simulink model "BLDC_system_diagram"  (R2013a)
settings: Solver=ode45  StartTime=0.0  StopTime=0.5  RelTol=1e-3
undefined symbols (not defined in the file or in its folder): Accelerationmax, Accelerationmin, DiscIntNeverNeededParam, IDCmax, IDCmin, Iphasepeakmax, P, PM, Risetimemax, Speedmax, Stalltimemax, Temperaturemax, Ts, VDCmax, VDCmin, VDCrated
undefined symbols (not defined in the file): Rs
libraries: simulink x68, powerlib_meascontrol x9, spsPMSynchronousMachineModel x3, simulink_extras x2
(part 1 of 3)
settings Model: Creator=Sony  LastModifiedBy=Muhammad Shamaas

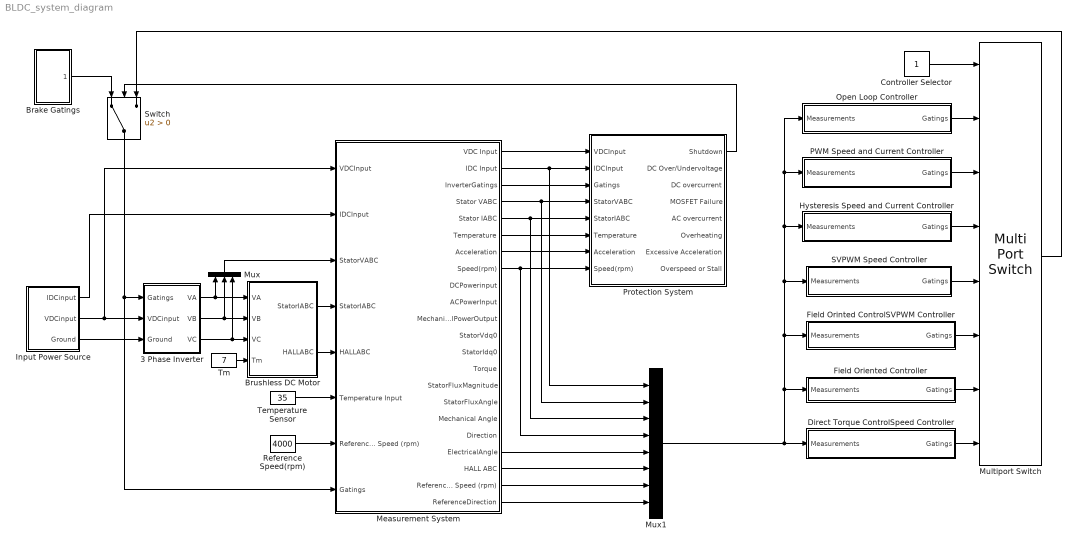
== system BLDC_system_diagram ==
  " Field Orinted ControlSVPWM Controller" : Subsystem
  3 Phase Inverter : Subsystem
  Brake Gatings : Subsystem
  Brushless DC Motor : Subsystem
  Controller Selector : Constant
  Direct Torque ControlSpeed Controller : Subsystem
  Field Oriented Controller : Subsystem
  Hysteresis Speed and Current Controller : Subsystem
  Input Power Source : Subsystem
  Measurement System : Subsystem
  Multiport Switch : MultiPortSwitch  Inputs=7
  Mux : Mux  Inputs=3
  Mux1 : Mux  Inputs=8
  Open Loop Controller : Subsystem
  PWM Speed and Current Controller : Subsystem
  Protection System : Subsystem
  Reference Speed(rpm) : Constant  Value=4000
  SVPWM Speed Controller : Subsystem
  Switch : Switch  Criteria=u2 > Threshold
  Temperature Sensor : Constant  Value=35
  Tm : Constant  Value=7
  wires:
  Input Power Source/2(VDCinput) -> Measurement System/1(VDCInput), 3 Phase Inverter/2(VDCinput)
  Input Power Source/3(Ground) -> 3 Phase Inverter/3(Ground)
  3 Phase Inverter/1(VA) -> Brushless DC Motor/1(VA), Mux/1
  3 Phase Inverter/2(VB) -> Brushless DC Motor/2(VB), Mux/2
  Brushless DC Motor/2(HALLABC) -> Measurement System/5(HALLABC)
  Brushless DC Motor/1(StatorIABC) -> Measurement System/4(StatorIABC)
  Mux/1 -> Measurement System/3(StatorVABC)
  3 Phase Inverter/3(VC) -> Brushless DC Motor/3(VC), Mux/3
  Measurement System/8(Speed(rpm)) -> Mux1/4, Protection System/8(Speed(rpm))
  Measurement System/7(Acceleration) -> Protection System/7(Acceleration)
  Measurement System/6(Temperature) -> Protection System/6(Temperature)
  Measurement System/5(Stator IABC) -> Mux1/3, Protection System/5(StatorIABC)
  Measurement System/4(Stator VABC) -> Mux1/2, Protection System/4(StatorVABC)
  Measurement System/3(InverterGatings) -> Protection System/3(Gatings)
  Measurement System/1(VDC Input) -> Protection System/1(VDCInput)
  Switch/1 -> Measurement System/8(Gatings), 3 Phase Inverter/1(Gatings)
  Multiport Switch/1 -> Switch/3
  Protection System/1(Shutdown) -> Switch/2
  Controller Selector/1 -> Multiport Switch/1
  Measurement System/2(IDC Input) -> Mux1/1, Protection System/2(IDCInput)
  Mux1/1 -> Field Oriented Controller/1(Measurements), " Field Orinted ControlSVPWM Controller"/1(Measurements), SVPWM Speed Controller/1(Measurements), Open Loop Controller/1(Measurements), PWM Speed and Current Controller/1(Measurements), Hysteresis Speed and Current Controller/1(Measurements), Direct Torque ControlSpeed Controller/1(Measurements)
  Measurement System/22(ReferenceDirection) -> Mux1/8
  Measurement System/21(Reference Speed (rpm)) -> Mux1/7
  Measurement System/20(HALL ABC) -> Mux1/6
  Measurement System/19(ElectricalAngle) -> Mux1/5
  Reference Speed(rpm)/1 -> Measurement System/7(Reference Speed (rpm))
  Brake Gatings/1(Gatings) -> Switch/1
  Open Loop Controller/1(Gatings) -> Multiport Switch/2
  PWM Speed and Current Controller/1(Gatings) -> Multiport Switch/3
  Hysteresis Speed and Current Controller/1(Gatings) -> Multiport Switch/4
  SVPWM Speed Controller/1(Gatings) -> Multiport Switch/5
  " Field Orinted ControlSVPWM Controller"/1(Gatings) -> Multiport Switch/6
  Field Oriented Controller/1(Gatings) -> Multiport Switch/7
  Direct Torque ControlSpeed Controller/1(Gatings) -> Multiport Switch/8
  Input Power Source/1(IDCinput) -> Measurement System/2(IDCInput)
  Temperature Sensor/1 -> Measurement System/6(Temperature Input)
  Tm/1 -> Brushless DC Motor/4(Tm)

== system BLDC_system_diagram/ Field Orinted ControlSVPWM Controller ==
  Measurements : Inport
  " Field Orinted ControlSVPWM Controller" : Subsystem
  Fcn14 : Fcn  Expr=u(5)
  Fcn15 : Fcn  Expr=u(7)
  Fcn16 : Fcn  Expr=u(3)
  Fcn17 : Fcn  Expr=u(4)
  Gatings : Outport
  wires:
  " Field Orinted ControlSVPWM Controller"/1(Gatings) -> Gatings/1
  Fcn14/1 -> " Field Orinted ControlSVPWM Controller"/4(Thetae)
  Fcn17/1 -> " Field Orinted ControlSVPWM Controller"/1(RotorSpeed(rpm))
  Fcn16/1 -> " Field Orinted ControlSVPWM Controller"/2(Iabc)
  Fcn15/1 -> " Field Orinted ControlSVPWM Controller"/3(ReferenceRotorSpeed(rpm))
  Measurements/1 -> Fcn14/1, Fcn15/1, Fcn17/1, Fcn16/1

== system BLDC_system_diagram/3 Phase Inverter ==
  note: Three Phase Inverter
      | HighSideGateSignal       LowSideGateSignal       Output
      | 0                                  0                 undefined
      | 0                                  1                    Ground
      | 1                                  0                 VDCInput
      | 1                                  1                   undefined
  Gatings : Inport
  VDCinput : Inport  Port=2
  Ground : Inport  Port=3
  Average : Subsystem
  Average1 : Subsystem
  Average2 : Subsystem
  Demux : Demux  Outputs=6
  Switch{,1..5} (6 alike) : Switch
  VA : Outport
  VB : Outport  Port=2
  VC : Outport  Port=3
  wires:
  [s1] -> Switch/2
  Demux/1 -> [s1]
  Demux/2 -> [s2]
  Demux/3 -> [s3]
  Demux/4 -> [s4]
  Demux/5 -> [s5]
  Demux/6 -> [s6]
  Gatings/1 -> Demux/1
  [s2] -> Switch3/2
  VDCinput/1 -> Switch/1, Switch5/1, Switch4/1
  Switch/1 -> Average/1(In1)
  Switch3/1 -> Average/2(In2)
  Average/1(Out1) -> VA/1
  Average1/1(Out1) -> VB/1
  Average2/1(Out1) -> VC/1
  [s4] -> Switch1/2
  [s6] -> Switch2/2
  Ground/1 -> Switch3/1, Switch2/1, Switch1/1
  [s3] -> Switch4/2
  [s5] -> Switch5/2
  Switch4/1 -> Average1/1(In1)
  Switch1/1 -> Average1/2(In2)
  Switch2/1 -> Average2/2(In2)
  Switch5/1 -> Average2/1(In1)

== system BLDC_system_diagram/Brake Gatings ==
  Brake Gatings : Constant  Value=[0;0;0]
  Compare To Zero : simulink/Logic and Bit Operations/Compare To Zero  relop=>=  OutDataTypeStr=boolean
  Constant : Constant  Value=0
  Gates : Subsystem
  Sum2 : Sum  Inputs=|+-
  TRI : powerlib_meascontrol/Pulse & Signal Generators/Triangle Generator  Freq=1e4  Phase=0  Ts=0
  Gatings : Outport
  wires:
  Compare To Zero/1 -> Gates/2(PWM)
  Gates/1(Gates) -> Gatings/1
  Sum2/1 -> Compare To Zero/1
  TRI/1 -> Sum2/2
  Brake Gatings/1 -> Gates/1("emf_abc ")
  Constant/1 -> Sum2/1

== system BLDC_system_diagram/Brushless DC Motor ==
  VA : Inport
  VB : Inport  Port=2
  VC : Inport  Port=3
  Tm : Inport  Port=4
  Add : Sum  Inputs=+-
  Add1 : Sum  Inputs=+-
  Electrical Model : Subsystem
  Mechanical Model : Subsystem
  Mux : Mux  Inputs=2
  Mux1 : Mux  Inputs=3
  Mux2 : Mux  Inputs=3
  Subsystem : Subsystem
  StatorIABC : Outport
  HALLABC : Outport  Port=2
  wires:
  Tm/1 -> Mechanical Model/1(Tm)
  Add/1 -> Mux/1
  Add1/1 -> Mux/2
  Mux/1 -> Electrical Model/1(v)  "vab,vbc"
  Electrical Model/1(m) -> Subsystem/1(m_e)
  Mechanical Model/2(the) -> Electrical Model/3(the)
  VB/1 -> Add1/1, Add/2
  VC/1 -> Add1/2
  Mechanical Model/1(we) -> Electrical Model/2(we)
  Electrical Model/2(Te) -> Mechanical Model/2(Te)
  Mechanical Model/3(m) -> Subsystem/2(m_m)
  VA/1 -> Add/1
  Subsystem/1(Stator current is_a (A)) -> Mux1/1
  Subsystem/2(Stator current is_b (A)) -> Mux1/2
  Subsystem/3(Stator current is_c (A)) -> Mux1/3
  Subsystem/4(Hall effect signal h_a) -> Mux2/1
  Subsystem/5(Hall effect signal h_b) -> Mux2/2
  Subsystem/6(Hall effect signal h_c) -> Mux2/3
  Mux2/1 -> HALLABC/1
  Mux1/1 -> StatorIABC/1

== system BLDC_system_diagram/Direct Torque ControlSpeed Controller ==
  Measurements : Inport
  Direct Torque ControlSpeed Controller : Subsystem
  Fcn22 : Fcn  Expr=u(7)
  Fcn23 : Fcn  Expr=u(4)
  Fcn24 : Fcn  Expr=u(3)
  Fcn25 : Fcn  Expr=u(2)
  Gatings : Outport
  wires:
  Direct Torque ControlSpeed Controller/1(Gatings) -> Gatings/1
  Fcn22/1 -> Direct Torque ControlSpeed Controller/4(ReferenceRotorSpeed(rpm))
  Fcn23/1 -> Direct Torque ControlSpeed Controller/3(RotorSpeed(rpm))
  Fcn24/1 -> Direct Torque ControlSpeed Controller/2(StatorIABC)
  Fcn25/1 -> Direct Torque ControlSpeed Controller/1(StatorVABC)
  Measurements/1 -> Fcn22/1, Fcn23/1, Fcn25/1, Fcn24/1

== system BLDC_system_diagram/Field Oriented Controller ==
  Measurements : Inport
  Fcn18 : Fcn  Expr=u(7)
  Fcn19 : Fcn  Expr=u(5)
  Fcn20 : Fcn  Expr=u(4)
  Fcn21 : Fcn  Expr=u(3)
  Field Oriented Control Current and Speed Controller : Subsystem
  Gatings : Outport
  wires:
  Field Oriented Control Current and Speed Controller/1(Gatings) -> Gatings/1
  Fcn20/1 -> Field Oriented Control Current and Speed Controller/2(RotorSpeed(rpm))
  Fcn19/1 -> Field Oriented Control Current and Speed Controller/3(Rotor Electrical Angle)
  Fcn21/1 -> Field Oriented Control Current and Speed Controller/1(Stator IABC)
  Fcn18/1 -> Field Oriented Control Current and Speed Controller/4(ReferenceRotorSpeed(rpm))
  Measurements/1 -> Fcn18/1, Fcn19/1, Fcn21/1, Fcn20/1

== system BLDC_system_diagram/Hysteresis Speed and Current Controller ==
  Measurements : Inport
  Fcn10 : Fcn  Expr=u(6)
  Fcn7 : Fcn  Expr=u(7)
  Fcn8 : Fcn  Expr=u(4)
  Fcn9 : Fcn  Expr=u(3)
  Hysteresis Speed and Current Controller : Subsystem
  Gatings : Outport
  wires:
  Measurements/1 -> Fcn7/1, Fcn8/1, Fcn10/1, Fcn9/1
  Fcn10/1 -> Hysteresis Speed and Current Controller/1(HALLABC)
  Hysteresis Speed and Current Controller/1(Gatings) -> Gatings/1
  Fcn8/1 -> Hysteresis Speed and Current Controller/3(RotorSpeed(rpm))
  Fcn7/1 -> Hysteresis Speed and Current Controller/4(ReferenceRotorSpeed(rpm))
  Fcn9/1 -> Hysteresis Speed and Current Controller/2(StatorIABC)

== system BLDC_system_diagram/Input Power Source ==
  IDCinput : Outport
  VDCinput : Outport  Port=2
  Ground : Outport  Port=3

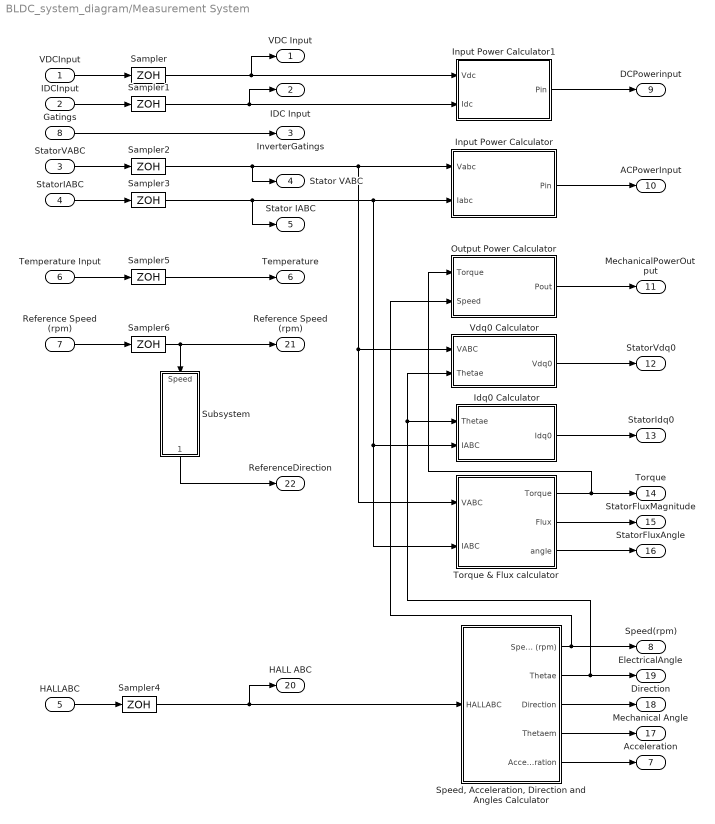
== system BLDC_system_diagram/Measurement System ==
  VDCInput : Inport
  IDCInput : Inport  Port=2
  StatorVABC : Inport  Port=3
  StatorIABC : Inport  Port=4
  HALLABC : Inport  Port=5
  Temperature Input : Inport  Port=6
  Reference Speed (rpm) : Inport  Port=7
  Gatings : Inport  Port=8
  Idq0 Calculator : Subsystem
  Input Power Calculator : Subsystem
  Input Power Calculator1 : Subsystem
  Output Power Calculator : Subsystem
  Sampler{,1..6} (7 alike) : ZeroOrderHold  SampleTime=1e-4
  "Speed, Acceleration, Direction and Angles Calculator" : Subsystem
  Subsystem : Subsystem
  Torque & Flux calculator : Subsystem  AncestorBlock=electricdrivelib/AC drives/DTC Induction Motor Drive/DTC/Torque & Flux calculator  mask{Rss=Rs, P=P, Ts=Ts}
  Vdq0 Calculator : Subsystem
  VDC Input : Outport
  IDC Input : Outport  Port=2
  InverterGatings : Outport  Port=3
  Stator VABC : Outport  Port=4
  Stator IABC : Outport  Port=5
  Temperature : Outport  Port=6
  Acceleration : Outport  Port=7
  Speed(rpm) : Outport  Port=8
  DCPowerinput : Outport  Port=9
  ACPowerInput : Outport  Port=10
  MechanicalPowerOutput : Outport  Port=11
  StatorVdq0 : Outport  Port=12
  StatorIdq0 : Outport  Port=13
  Torque : Outport  Port=14
  StatorFluxMagnitude : Outport  Port=15
  StatorFluxAngle : Outport  Port=16
  Mechanical Angle : Outport  Port=17
  Direction : Outport  Port=18
  ElectricalAngle : Outport  Port=19
  HALL ABC : Outport  Port=20
  Reference Speed (rpm) : Outport  Port=21
  ReferenceDirection : Outport  Port=22
  wires:
  HALLABC/1 -> Sampler4/1
  Sampler/1 -> VDC Input/1, Input Power Calculator1/1(Vdc)
  IDCInput/1 -> Sampler1/1
  "Speed, Acceleration, Direction and Angles Calculator"/2(Thetae) -> ElectricalAngle/1, Idq0 Calculator/1(Thetae), Vdq0 Calculator/2(Thetae)
  StatorIABC/1 -> Sampler3/1
  Torque & Flux calculator/1(Torque) -> Torque/1, Output Power Calculator/1(Torque)
  StatorVABC/1 -> Sampler2/1
  "Speed, Acceleration, Direction and Angles Calculator"/1(Speed (rpm)) -> Output Power Calculator/2(Speed), Speed(rpm)/1
  Input Power Calculator1/1(Pin) -> DCPowerinput/1
  Torque & Flux calculator/3(angle) -> StatorFluxAngle/1
  "Speed, Acceleration, Direction and Angles Calculator"/5(Acceleration) -> Acceleration/1
  Output Power Calculator/1(Pout) -> MechanicalPowerOutput/1
  Idq0 Calculator/1(Idq0) -> StatorIdq0/1
  "Speed, Acceleration, Direction and Angles Calculator"/3(Direction) -> Direction/1
  Input Power Calculator/1(Pin) -> ACPowerInput/1
  Vdq0 Calculator/1(Vdq0) -> StatorVdq0/1
  "Speed, Acceleration, Direction and Angles Calculator"/4(Thetaem) -> Mechanical Angle/1
  Torque & Flux calculator/2(Flux) -> StatorFluxMagnitude/1
  VDCInput/1 -> Sampler/1
  Sampler1/1 -> IDC Input/1, Input Power Calculator1/2(Idc)
  Sampler2/1 -> Stator VABC/1, Torque & Flux calculator/1(VABC), Vdq0 Calculator/1(VABC), Input Power Calculator/1(Vabc)
  Sampler3/1 -> Stator IABC/1, Torque & Flux calculator/2(IABC), Idq0 Calculator/2(IABC), Input Power Calculator/2(Iabc)
  Sampler4/1 -> HALL ABC/1, "Speed, Acceleration, Direction and Angles Calculator"/1(HALLABC)
  Temperature Input/1 -> Sampler5/1
  Sampler5/1 -> Temperature/1
  Reference Speed (rpm)/1 -> Sampler6/1
  Sampler6/1 -> Subsystem/1(Speed), Reference Speed (rpm)/1
  Gatings/1 -> InverterGatings/1
  Subsystem/1(Direction) -> ReferenceDirection/1

== system BLDC_system_diagram/Open Loop Controller ==
  Measurements : Inport
  Fcn : Fcn  Expr=u(6)
  Fcn1 : Fcn  Expr=u(8)
  Open Loop Controller : Subsystem
  Gatings : Outport
  wires:
  Open Loop Controller/1(Gatings) -> Gatings/1
  Fcn1/1 -> Open Loop Controller/2(Direction)
  Fcn/1 -> Open Loop Controller/1(HALLSensorABCSignals)
  Measurements/1 -> Fcn1/1, Fcn/1

== system BLDC_system_diagram/PWM Speed and Current Controller ==
  Measurements : Inport
  Fcn2 : Fcn  Expr=u(7)
  Fcn4 : Fcn  Expr=u(4)
  Fcn5 : Fcn  Expr=u(1)
  Fcn6 : Fcn  Expr=u(6)
  PWM Speed and Current Controller : Subsystem
  Gatings : Outport
  wires:
  Fcn6/1 -> PWM Speed and Current Controller/1(HALLABC)
  Fcn5/1 -> PWM Speed and Current Controller/2(IDCInput)
  Fcn4/1 -> PWM Speed and Current Controller/3(RotorSpeed(rpm))
  Fcn2/1 -> PWM Speed and Current Controller/4(ReferenceRotorSpeed(rpm))
  PWM Speed and Current Controller/1(Gatings) -> Gatings/1
  Measurements/1 -> Fcn2/1, Fcn4/1, Fcn6/1, Fcn5/1

== system BLDC_system_diagram/Protection System ==
  VDCInput : Inport
  IDCInput : Inport  Port=2
  Gatings : Inport  Port=3
  StatorVABC : Inport  Port=4
  StatorIABC : Inport  Port=5
  Temperature : Inport  Port=6
  Acceleration : Inport  Port=7
  Speed(rpm) : Inport  Port=8
  AC overcurrent Protection : Subsystem
  DC Over/Undervoltage Protection : Subsystem
  DC overcurrent Protection : Subsystem
  Excessive Acceleration/Deceleration Protection : Subsystem
  Logical Operator : Logic  Operator=OR  Inputs=7  AllPortsSameDT=off  OutDataTypeStr=boolean
  MOSFET Failure Protection : Subsystem
  Overheating Protection : Subsystem
  Overspeed and Stall Protection : Subsystem
  Shutdown : Outport
  DC Over/Undervoltage : Outport  Port=2
  DC overcurrent : Outport  Port=3
  MOSFET Failure : Outport  Port=4
  AC overcurrent : Outport  Port=5
  Overheating : Outport  Port=6
  Excessive Acceleration : Outport  Port=7
  Overspeed or Stall : Outport  Port=8
  tag scope: Shutdown=global
  wires:
  AC overcurrent Protection/1(Out1) -> Logical Operator/4, AC overcurrent/1
  DC overcurrent Protection/1(Out1) -> Logical Operator/2, DC overcurrent/1
  DC Over/Undervoltage Protection/1(Out1) -> Logical Operator/1, DC Over/Undervoltage/1
  Overheating Protection/1(Out1) -> Logical Operator/5, Overheating/1
  MOSFET Failure Protection/1(Out1) -> Logical Operator/3, MOSFET Failure/1
  Excessive Acceleration/Deceleration Protection/1(Out1) -> Logical Operator/6, Excessive Acceleration/1
  Overspeed and Stall Protection/1(Out1) -> Logical Operator/7, Overspeed or Stall/1
  Logical Operator/1 -> [Shutdown], Shutdown/1
  VDCInput/1 -> DC Over/Undervoltage Protection/1(VDC)
  IDCInput/1 -> DC overcurrent Protection/1(IDCInput)
  Gatings/1 -> MOSFET Failure Protection/1(Gatings)
  StatorVABC/1 -> MOSFET Failure Protection/2(StatorVABC)
  StatorIABC/1 -> AC overcurrent Protection/1(StatorIABC)
  Temperature/1 -> Overheating Protection/1(Temperature)
  Acceleration/1 -> Excessive Acceleration/Deceleration Protection/1(Acceleration)
  Speed(rpm)/1 -> Overspeed and Stall Protection/1(Speed(rpm))

== system BLDC_system_diagram/SVPWM Speed Controller ==
  Measurements : Inport
  Fcn11 : Fcn  Expr=u(7)
  Fcn12 : Fcn  Expr=u(4)
  Fcn13 : Fcn  Expr=u(6)
  SVPWM Speed Controller : Subsystem
  Gatings : Outport
  wires:
  SVPWM Speed Controller/1(Gatings) -> Gatings/1
  Fcn13/1 -> SVPWM Speed Controller/1(HALLABC)
  Fcn12/1 -> SVPWM Speed Controller/2(RotorSpeed(rpm))
  Fcn11/1 -> SVPWM Speed Controller/3(ReferenceRotorSpeed(rpm))
  Measurements/1 -> Fcn11/1, Fcn13/1, Fcn12/1

== system BLDC_system_diagram/ Field Orinted ControlSVPWM Controller/ Field Orinted ControlSVPWM Controller ==
  note: void writestate (int sa, int sb, int sc)
      | {
      |   if (sa==1)    {digitalWrite(PhaseaUpperPin, HIGH);digitalWrite(PhaseaLowerPin, LOW);}
      |   if (sa==(-1)){digitalWrite(PhaseaUpperPin, LOW) ;digitalWrite(PhaseaLowerPin, HIGH);}
      |   if (sa==0)    {digitalWrite(PhaseaUpperPin, LOW) ;digitalWrite(PhaseaLowerPin, LOW);}
      |   if (sb==1)    {digitalWrite(PhasebUpperPin, HIGH);digitalWrite(PhasebLowerPin, LOW);}
      |   if (sb==(-1)){digitalWrite(PhasebUpperPin, LOW) ;digitalWrite(PhasebLowerPin, HIGH);}
      |   if (sb==0)    {digitalWrite(PhasebUpperPin, LOW) ;digitalWrite(PhasebLowerPin, LOW);}
      |   if (sc==1)    {digitalWrite(PhasecUpperPin, HIGH);digitalWrite(PhasecLowerPin, LOW);}
      |   if (sc==(-1)){digitalWrite(PhasecUpperPin, LOW) ;digitalWrite(PhasecLowerPin, HIGH);}
      |   if (sc==0)    {digitalWrite(PhasecUpperPin, LOW) ;digitalWrite(PhasecLowerPin, LOW);}
      | }
      |
      | void loop()
      | {
      |
      |   IA=analogRead(IaPin);
      |   IB=analogRead(IbPin);
      |   IC=analogRead(IcPin);
      |
      |   Ialpha=(2/3)*((1)  *IA+(-1/2)     *IB+(-1/2)      *IC);
      |   Ibeta =(2/3)*((0)  *IA+(sqrt(3)/2)*IB+(-sqrt(3)/2)*IC);
      |   I0=    (2/3)*((1/2)*IA+(1/2)      *IB+(1/2)       *IC);
      |
      |   Id=Ialpha*( cos(thetae))+Ibeta*(sin(thetae));
      |   Iq=Ialpha*(-sin(thetae))+Ibeta*(cos(thetae));
      |
      |   Speedref=analogRead(SpeedrefPin);
      |   SpeedErrorOld=SpeedErrorNew;
      |   SpeedErrorNew=newspeed-Speedref;
      |   Iqref=kps*SpeedErrorNew+kis*(0.5)*(SpeedErrorNew+SpeedErrorOld)*Ts;
      |   Idref=0;
      |   I0ref=0;
      |
      |   IqErrorOld=IqErrorNew;
      |   IdErrorOld=IqErrorNew;
      |   IqErrorNew=Iq-Iqref;
      |   IdErrorNew=Id-Idref;
      |   Vd=kp*IdErrorNew+ki*(0.5)*(IdErrorNew+IdErrorOld)*Ts;
      |   Vq=kp*IqErrorNew+ki*(0.5)*(IqErrorNew+IqErrorOld)*Ts;;
      |   vref=sqrt(Vd*Vd+Vq*Vq);
      |
      |   sector=(thetae/(PI/3))+1;
      |   thetae=thetae-(sector-1)*(PI/3);
      |
      |   T1=sqrt(3)*Ts*vref*(1/Vdc)*sin((PI/3)-thetae);
      |   T2=sqrt(3)*Ts*vref*(1/Vdc)*sin(thetae);
      |   T0=Ts-T1-T2;
      |
      |
      |
      |   if (sector==1)
      |   {
      |     writeState(B000);delayMicroseconds(T0/2);
      |     writeState(B100);delayMicroseconds(T1);
      |     writeState(B110);delayMicroseconds(T2);
      |     writeState(B111);delayMicroseconds(T0);
      |     writeState(B110);delayMicroseconds(T2);
      |     writeState(B100);delayMicroseconds(T1);
      |     writeState(B000);delayMicroseconds(T0/2);
      |   }
      |
      |   if (sector==2)
      |   {
      |     writeState(B000);delayMicroseconds(T0/2);
      |     writeState(B010);delayMicroseconds(T2);
      |     writeState(B110);delayMicroseconds(T1);
      |     writeState(B111);delayMicroseconds(T0);
      |     writeState(B110);delayMicroseconds(T1);
      |     writeState(B010);delayMicroseconds(T2);
      |     writeState(B000);delayMicroseconds(T0/2);
      |   }
      |
      |   if (sector==3)
      |   {
      |     writeState(B000);delayMicroseconds(T0/2);
      |     writeState(B010);delayMicroseconds(T1);
      |     writeState(B011);delayMicroseconds(T2);
      |     writeState(B111);delayMicroseconds(T0);
      |     writeState(B011);delayMicroseconds(T2);
      |     writeState(B010);delayMicroseconds(T1);
      |     writeState(B000);delayMicroseconds(T0/2);
      |   }
      |
      |   if (sector==4)
      |   {
      |     writeState(B000);delayMicroseconds(T0/2);
      |     writeState(B001);delayMicroseconds(T2);
      |     writeState(B011);delayMicroseconds(T1);
      |     writeState(B111);delayMicroseconds(T0);
      |     writeState(B011);delayMicroseconds(T1);
      |     writeState(B001);delayMicroseconds(T2);
      |     writeState(B000);delayMicroseconds(T0/2);
      |   }
      |
      |   if (sector==5)
      |   {
      |     writeState(B000);delayMicroseconds(T0/2);
      |     writeState(B001);delayMicroseconds(T1);
      |     writeState(B101);delayMicroseconds(T2);
      |     writeState(B111);delayMicroseconds(T0);
      |     writeState(B101);delayMicroseconds(T2);
      |     writeState(B001);delayMicroseconds(T1);
      |     writeState(B000);delayMicroseconds(T0/2);
      |   }
      |
      |   if (sector==6)
      |   {
      |     writeState(B000);delayMicroseconds(T0/2);
      |     writeState(B001);delayMicroseconds(T2);
      |     writeState(B011);delayMicroseconds(T1);
      |     writeState(B111);delayMicroseconds(T0);
      |     writeState(B011);delayMicroseconds(T1);
      |     writeState(B001);delayMicroseconds(T2);
      |     writeState(B000);delayMicroseconds(T0/2);
      |   }
      | }
  note: iq
  note: id
  note: vabc
  note: vdq0
  note: vq_ref
  note: vd_ref
  note: iq_ref
  RotorSpeed(rpm) : Inport
  Iabc : Inport  Port=2
  ReferenceRotorSpeed(rpm) : Inport  Port=3
  Thetae : Inport  Port=4
  Demux : Demux  Outputs=3
  Mux1 : Mux  Inputs=3
  PID Controller : simulink/Continuous/PID Controller  Controller=PID  TimeDomain=Continuous-time  SampleTime=1  IntegratorMethod=Forward Euler  FilterMethod=Forward Euler  Form=Parallel  P=0.005  I=0.100  D=0  N=100  InitialConditionSource=internal  InitialConditionForIntegrator=0  InitialConditionForFilter=0  ExternalReset=none  LimitOutput=on  UpperSaturationLimit=125  LowerSaturationLimit=-125  LinearizeAsGain=on  AntiWindupMode=none  Kb=1  TrackingMode=off  Kt=1  PParamMin=[]  PParamMax=[]  IParamMin=[]  IParamMax=[]  DParamMin=[]  DParamMax=[]  NParamMin=[]  NParamMax=[]  KbParamMin=[]  KbParamMax=[]  KtParamMin=[]  KtParamMax=[]  POutMin=[]  POutMax=[]  IOutMin=[]  IOutMax=[]  DOutMin=[]  DOutMax=[]  NOutMin=[]  NOutMax=[]  KbOutMin=[]  KbOutMax=[]  KtOutMin=[]  KtOutMax=[]  IntegratorOutMin=[]  IntegratorOutMax=[]  FilterOutMin=[]  FilterOutMax=[]  SumOutMin=[]  SumOutMax=[]  SumI1OutMin=[]  SumI1OutMax=[]  SumI2OutMin=[]  SumI2OutMax=[]  SumI3OutMin=[]  SumI3OutMax=[]  SumDOutMin=[]  SumDOutMax=[]  SaturationOutMin=[]  SaturationOutMax=[]  IntegratorContinuousStateAttributes=''  IntegratorStateMustResolveToSignalObject=off  IntegratorRTWStateStorageClass=Auto  FilterContinuousStateAttributes=''  FilterStateMustResolveToSignalObject=off  FilterRTWStateStorageClass=Auto
  PID Controller1 : simulink/Continuous/PID Controller  Controller=PID  TimeDomain=Continuous-time  SampleTime=1  IntegratorMethod=Forward Euler  FilterMethod=Forward Euler  Form=Parallel  P=0.5  I=1  D=0  N=100  InitialConditionSource=internal  InitialConditionForIntegrator=0  InitialConditionForFilter=0  ExternalReset=none  LimitOutput=on  UpperSaturationLimit=48/2  LowerSaturationLimit=-48/2  LinearizeAsGain=on  AntiWindupMode=none  Kb=1  TrackingMode=off  Kt=1  PParamMin=[]  PParamMax=[]  IParamMin=[]  IParamMax=[]  DParamMin=[]  DParamMax=[]  NParamMin=[]  NParamMax=[]  KbParamMin=[]  KbParamMax=[]  KtParamMin=[]  KtParamMax=[]  POutMin=[]  POutMax=[]  IOutMin=[]  IOutMax=[]  DOutMin=[]  DOutMax=[]  NOutMin=[]  NOutMax=[]  KbOutMin=[]  KbOutMax=[]  KtOutMin=[]  KtOutMax=[]  IntegratorOutMin=[]  IntegratorOutMax=[]  FilterOutMin=[]  FilterOutMax=[]  SumOutMin=[]  SumOutMax=[]  SumI1OutMin=[]  SumI1OutMax=[]  SumI2OutMin=[]  SumI2OutMax=[]  SumI3OutMin=[]  SumI3OutMax=[]  SumDOutMin=[]  SumDOutMax=[]  SaturationOutMin=[]  SaturationOutMax=[]  IntegratorContinuousStateAttributes=''  IntegratorStateMustResolveToSignalObject=off  IntegratorRTWStateStorageClass=Auto  FilterContinuousStateAttributes=''  FilterStateMustResolveToSignalObject=off  FilterRTWStateStorageClass=Auto
  PID Controller2 : simulink/Continuous/PID Controller  Controller=PID  TimeDomain=Continuous-time  SampleTime=1  IntegratorMethod=Forward Euler  FilterMethod=Forward Euler  Form=Parallel  P=0.5  I=1  D=0  N=100  InitialConditionSource=internal  InitialConditionForIntegrator=0  InitialConditionForFilter=0  ExternalReset=none  LimitOutput=on  UpperSaturationLimit=48/2  LowerSaturationLimit=-48/2  LinearizeAsGain=on  AntiWindupMode=none  Kb=1  TrackingMode=off  Kt=1  PParamMin=[]  PParamMax=[]  IParamMin=[]  IParamMax=[]  DParamMin=[]  DParamMax=[]  NParamMin=[]  NParamMax=[]  KbParamMin=[]  KbParamMax=[]  KtParamMin=[]  KtParamMax=[]  POutMin=[]  POutMax=[]  IOutMin=[]  IOutMax=[]  DOutMin=[]  DOutMax=[]  NOutMin=[]  NOutMax=[]  KbOutMin=[]  KbOutMax=[]  KtOutMin=[]  KtOutMax=[]  IntegratorOutMin=[]  IntegratorOutMax=[]  FilterOutMin=[]  FilterOutMax=[]  SumOutMin=[]  SumOutMax=[]  SumI1OutMin=[]  SumI1OutMax=[]  SumI2OutMin=[]  SumI2OutMax=[]  SumI3OutMin=[]  SumI3OutMax=[]  SumDOutMin=[]  SumDOutMax=[]  SaturationOutMin=[]  SaturationOutMax=[]  IntegratorContinuousStateAttributes=''  IntegratorStateMustResolveToSignalObject=off  IntegratorRTWStateStorageClass=Auto  FilterContinuousStateAttributes=''  FilterStateMustResolveToSignalObject=off  FilterRTWStateStorageClass=Auto
  SVPWM : Subsystem  mask{Fs=10000, Fsampling=10000, Vbase=48/2, Vdc=48/2}
  Sum : Sum  Inputs=|+-
  Sum1 : Sum  Inputs=|+-
  Sum2 : Sum  Inputs=|+-
  abc to dq0 : powerlib_meascontrol/Transformations/abc to dq0  Alignment=Aligned with phase A axis
  dq0 to abc : powerlib_meascontrol/Transformations/dq0 to abc  Alignment=Aligned with phase A axis
  id_ref : Constant  Value=0
  v0 : Constant  Value=0
  Gatings : Outport
  wires:
  Sum/1 -> PID Controller/1
  abc to dq0/1 -> Demux/1
  PID Controller/1 -> Sum1/1
  id_ref/1 -> Sum2/1
  Demux/1 -> Sum2/2
  Demux/2 -> Sum1/2
  Sum1/1 -> PID Controller1/1
  Sum2/1 -> PID Controller2/1
  dq0 to abc/1 -> SVPWM/1(Vabc)
  Mux1/1 -> dq0 to abc/1
  PID Controller2/1 -> Mux1/1
  PID Controller1/1 -> Mux1/2
  Thetae/1 -> abc to dq0/2, dq0 to abc/2
  v0/1 -> Mux1/3
  RotorSpeed(rpm)/1 -> Sum/2
  Iabc/1 -> abc to dq0/1
  ReferenceRotorSpeed(rpm)/1 -> Sum/1
  SVPWM/1(Gatings) -> Gatings/1

== system BLDC_system_diagram/3 Phase Inverter/Average ==
  In1 : Inport
  In2 : Inport  Port=2
  Constant : Constant  Value=2
  Divide : Product  Inputs=*/
  netsum : Sum  Inputs=2  SaturateOnIntegerOverflow=on  InputSameDT=on  OutDataTypeStr=Inherit: Same as first input
  Out1 : Outport
  wires:
  In1/1 -> netsum/1
  Constant/1 -> Divide/2
  Divide/1 -> Out1/1
  In2/1 -> netsum/2
  netsum/1 -> Divide/1

== system BLDC_system_diagram/3 Phase Inverter/Average1 ==
  In1 : Inport
  In2 : Inport  Port=2
  Constant : Constant  Value=2
  Divide : Product  Inputs=*/
  netsum : Sum  Inputs=2  SaturateOnIntegerOverflow=on  InputSameDT=on  OutDataTypeStr=Inherit: Same as first input
  Out1 : Outport
  wires:
  In1/1 -> netsum/1
  Constant/1 -> Divide/2
  Divide/1 -> Out1/1
  In2/1 -> netsum/2
  netsum/1 -> Divide/1

== system BLDC_system_diagram/3 Phase Inverter/Average2 ==
  In1 : Inport
  In2 : Inport  Port=2
  Constant : Constant  Value=2
  Divide : Product  Inputs=*/
  netsum : Sum  Inputs=2  SaturateOnIntegerOverflow=on  InputSameDT=on  OutDataTypeStr=Inherit: Same as first input
  Out1 : Outport
  wires:
  In1/1 -> netsum/1
  Constant/1 -> Divide/2
  Divide/1 -> Out1/1
  In2/1 -> netsum/2
  netsum/1 -> Divide/1

== system BLDC_system_diagram/Brake Gatings/Gates ==
  note: This module implements the following true table
      |
      |    emf_a   |   emf_b   |   emf_c   ||   Q1   |   Q2   |   Q3   |   Q4   |   Q5   |   Q6
      |     ------------------------------------------------------------------------------------------------------------------
      |       0              0                0            0          0          0           0        0        0
      |       0               -1              +1          0          0          0           1        1        0
      |     -1              +1                0          0          1          1           0        0        0
      |     -1               0               +1          0          1         0           0        1        0
      |    +1               0                -1          1          0          0           0        0        1
      |    +1              -1                0           1          0          0           1        0        0
      |      0              +1               -1           0          0          1           0        0        1
      |     0              0                0             0          0          0           0        0        0
  "emf_abc " : Inport
  PWM : Inport  Port=2
  Compare To Zero : simulink/Logic and Bit Operations/Compare To Zero  relop=>  OutDataTypeStr=boolean  ZeroCross=off
  Compare To Zero2 : simulink/Logic and Bit Operations/Compare To Zero  relop=>  OutDataTypeStr=boolean  ZeroCross=off
  Compare To Zero4 : simulink/Logic and Bit Operations/Compare To Zero  relop=>  OutDataTypeStr=boolean  ZeroCross=off
  Demux2 : Demux  Outputs=3
  LO{,1..5} (6 alike) : Logic  AllPortsSameDT=off  OutDataTypeStr=boolean
  LO6 : Logic  Operator=NOT  AllPortsSameDT=off  OutDataTypeStr=boolean
  LO7 : Logic  Operator=NOT  AllPortsSameDT=off  OutDataTypeStr=boolean
  LO8 : Logic  Operator=NOT  AllPortsSameDT=off  OutDataTypeStr=boolean
  Mux3 : Mux  Inputs=6
  Gates : Outport
  wires:
  "emf_abc "/1 -> Demux2/1
  Mux3/1 -> Gates/1
  Demux2/1 -> Compare To Zero/1
  Demux2/2 -> Compare To Zero2/1
  Demux2/3 -> Compare To Zero4/1
  LO/1 -> Mux3/1
  LO6/1 -> LO1/2
  Compare To Zero/1 -> LO6/1, LO/2
  PWM/1 -> LO/1, LO5/1, LO4/1, LO3/1, LO2/1, LO1/1
  LO1/1 -> Mux3/2
  Compare To Zero2/1 -> LO7/1, LO2/2
  LO2/1 -> Mux3/3
  LO7/1 -> LO3/2
  Compare To Zero4/1 -> LO8/1, LO4/2
  LO8/1 -> LO5/2
  LO5/1 -> Mux3/6
  LO4/1 -> Mux3/5
  LO3/1 -> Mux3/4

== system BLDC_system_diagram/Brushless DC Motor/Electrical Model ==
  v : Inport
  we : Inport  Port=2
  the : Inport  Port=3
  "BEMF, Flux" : spsPMSynchronousMachineModel/Continuous Trapezoidal/BEMF, Flux
  Gain3 : Gain  Gain=PM.p  SaturateOnIntegerOverflow=on  OutDataTypeStr=Inherit: Same as input  ParamDataTypeStr=Inherit: Same as input
  Hall effect sensor : spsPMSynchronousMachineModel/Continuous Trapezoidal/Hall effect sensor
  Mux : Mux  Inputs=3
  Mux1 : Mux  Inputs=2
  Product : Product  SaturateOnIntegerOverflow=on  OutDataTypeStr=Inherit: Same as first input
  Selector : Selector  InputPortWidth=3  IndexOptions=Index vector (dialog)  Indices=1:2  OutputSizes=1
  State equations : spsPMSynchronousMachineModel/Continuous Trapezoidal/State equations
  Sum2 : Sum  Inputs=+  SaturateOnIntegerOverflow=on
  Terminator : Terminator
  m : Outport  InitialOutput=0
  Te : Outport  Port=2  InitialOutput=0
  wires:
  "BEMF, Flux"/1 -> Mux/2, State equations/2
  Gain3/1 -> Te/1
  Selector/1 -> Terminator/1
  we/1 -> Mux1/2
  Mux/1 -> m/1
  Hall effect sensor/1 -> Mux/3
  Product/1 -> Sum2/1
  Sum2/1 -> Gain3/1
  the/1 -> Hall effect sensor/1, Mux1/1
  State equations/1 -> Mux/1, Product/1, Selector/1
  Mux1/1 -> "BEMF, Flux"/1
  "BEMF, Flux"/2 -> Product/2
  v/1 -> State equations/1  "vab,vbc"

== system BLDC_system_diagram/Brushless DC Motor/Mechanical Model ==
  Tm : Inport
  Te : Inport  Port=2
  Coulomb & Viscous Friction : simulink/Discontinuities/Coulomb & Viscous Friction  offset=PM.Tf  gain=PM.F
  Fcn : Fcn  Expr=(u(1)-PM.thOffest)/PM.p
  Gain : Gain  Gain=PM.p  SaturateOnIntegerOverflow=on  OutDataTypeStr=Inherit: Same as input  ParamDataTypeStr=Inherit: Same as input
  Gain2 : Gain  Gain=1/PM.J  SaturateOnIntegerOverflow=on  OutDataTypeStr=Inherit: Same as input  ParamDataTypeStr=Inherit: Same as input
  Int : Integrator  InitialCondition=PM.wmo
  Int1 : Integrator  InitialCondition=PM.tho+PM.thOffest
  Mux1 : Mux  Inputs=3
  Sum : Sum  Inputs=-+-  SaturateOnIntegerOverflow=on  InputSameDT=on  OutDataTypeStr=Inherit: Same as first input
  we : Outport  InitialOutput=0
  the : Outport  Port=2  InitialOutput=0
  m : Outport  Port=3  InitialOutput=0
  wires:
  Fcn/1 -> Mux1/2
  Coulomb & Viscous Friction/1 -> Sum/3
  Mux1/1 -> m/1
  Tm/1 -> Sum/1
  Int1/1 -> the/1, Fcn/1
  Gain2/1 -> Int/1
  Gain/1 -> we/1, Int1/1
  Sum/1 -> Gain2/1
  Int/1 -> Gain/1, Coulomb & Viscous Friction/1, Mux1/1
  Te/1 -> Sum/2, Mux1/3

== system BLDC_system_diagram/Brushless DC Motor/Subsystem ==
  m_e : Inport
  m_m : Inport  Port=2
  Demux : Demux  Outputs=[1,1,1,1,1,1,1,1,1]
  Demux1 : Demux  Outputs=[1,1,1]
  Stator current is_a (A) : Outport
  Stator current is_b (A) : Outport  Port=2
  Stator current is_c (A) : Outport  Port=3
  Hall effect signal h_a : Outport  Port=4
  Hall effect signal h_b : Outport  Port=5
  Hall effect signal h_c : Outport  Port=6
  wires:
  m_m/1 -> Demux1/1
  Demux/3 -> Stator current is_c (A)/1  "Stator current is_c (A)"
  Demux/1 -> Stator current is_a (A)/1  "Stator current is_a (A)"
  Demux/2 -> Stator current is_b (A)/1  "Stator current is_b (A)"
  Demux/9 -> Hall effect signal h_c/1  "Hall effect signal h_c"
  Demux/8 -> Hall effect signal h_b/1  "Hall effect signal h_b"
  Demux/7 -> Hall effect signal h_a/1  "Hall effect signal h_a"
  m_e/1 -> Demux/1

== system BLDC_system_diagram/Direct Torque ControlSpeed Controller/Direct Torque ControlSpeed Controller ==
  StatorVABC : Inport
  StatorIABC : Inport  Port=2
  RotorSpeed(rpm) : Inport  Port=3
  ReferenceRotorSpeed(rpm) : Inport  Port=4
  -dTe/2 : Relay  OnSwitchValue=0  OffSwitchValue=-1/20000  OnOutputValue=0  OffOutputValue=3
  Data Type Conversion5 : DataTypeConversion  SaturateOnIntegerOverflow=on  RndMeth=Zero
  Flux sector seeker : Subsystem  AncestorBlock=electricdrivelib/AC drives/DTC Induction Motor Drive/DTC/Flux sector seeker
  Flux table : Subsystem  AncestorBlock=DriveInternalModels/AC drives/Speed Controller AC345/Speed Controller/Flux table  mask{bs=5000, nf=0.01}
      mask prompts: bs "Rated Speed (rpm)"; nf "Rated Stator Flux (Wb)"
      mask Display: plot([0;1800;2000;2500;3000;3500], [1;1;0.90*1;0.72*1;0.6*1;0.51*1])
  Gain : Gain  Gain=2  SaturateOnIntegerOverflow=on  OutDataTypeStr=Inherit: Same as input  ParamDataTypeStr=Inherit: Same as input
  Logical Operator : Logic  Operator=NOR  AllPortsSameDT=off
  PID Controller : simulink/Continuous/PID Controller  Controller=PID  TimeDomain=Continuous-time  SampleTime=1  IntegratorMethod=Forward Euler  FilterMethod=Forward Euler  Form=Parallel  P=0.0001  I=0.001  D=0  N=100  InitialConditionSource=internal  InitialConditionForIntegrator=0  InitialConditionForFilter=0  ExternalReset=none  LimitOutput=on  UpperSaturationLimit=20  LowerSaturationLimit=-20  LinearizeAsGain=on  AntiWindupMode=none  Kb=1  TrackingMode=off  Kt=1  PParamMin=[]  PParamMax=[]  IParamMin=[]  IParamMax=[]  DParamMin=[]  DParamMax=[]  NParamMin=[]  NParamMax=[]  KbParamMin=[]  KbParamMax=[]  KtParamMin=[]  KtParamMax=[]  POutMin=[]  POutMax=[]  IOutMin=[]  IOutMax=[]  DOutMin=[]  DOutMax=[]  NOutMin=[]  NOutMax=[]  KbOutMin=[]  KbOutMax=[]  KtOutMin=[]  KtOutMax=[]  IntegratorOutMin=[]  IntegratorOutMax=[]  FilterOutMin=[]  FilterOutMax=[]  SumOutMin=[]  SumOutMax=[]  SumI1OutMin=[]  SumI1OutMax=[]  SumI2OutMin=[]  SumI2OutMax=[]  SumI3OutMin=[]  SumI3OutMax=[]  SumDOutMin=[]  SumDOutMax=[]  SaturationOutMin=[]  SaturationOutMax=[]  IntegratorContinuousStateAttributes=''  IntegratorStateMustResolveToSignalObject=off  IntegratorRTWStateStorageClass=Auto  FilterContinuousStateAttributes=''  FilterStateMustResolveToSignalObject=off  FilterRTWStateStorageClass=Auto
  Sum : Sum  Inputs=|+-
  Sum1 : Sum  Inputs=|+-  SaturateOnIntegerOverflow=on
  Sum2 : Sum  Inputs=|+-  SaturateOnIntegerOverflow=on
  Sum3 : Sum  Inputs=+++  SaturateOnIntegerOverflow=on
  Switching table : Subsystem  AncestorBlock=electricdrivelib/AC drives/DTC Induction Motor Drive/DTC/Switching table
  Torque & Flux calculator : Subsystem  AncestorBlock=electricdrivelib/AC drives/DTC Induction Motor Drive/DTC/Torque & Flux calculator  mask{Rss=0.01, P=4, Ts=1/(10000)}
  dPhi : Relay  OnSwitchValue=1/20000  OffSwitchValue=-1/20000  OffOutputValue=2
  dTe/2 : Relay  OnSwitchValue=1/20000  OffSwitchValue=0
  Gatings : Outport
  wires:
  Torque & Flux calculator/1(Torque) -> Sum1/2
  Flux sector seeker/1(sector) -> Switching table/3(Sector)
  dPhi/1 -> Switching table/2(H Phi)
  Torque & Flux calculator/2(Flux) -> Sum2/2
  Switching table/1(Gates) -> Gatings/1
  Torque & Flux calculator/3(angle) -> Flux sector seeker/1(Flux_angle)
  Flux table/1(Flux) -> Sum2/1
  Sum3/1 -> Switching table/1(H Te)
  Sum/1 -> PID Controller/1
  ReferenceRotorSpeed(rpm)/1 -> Sum/1
  Sum2/1 -> dPhi/1
  StatorVABC/1 -> Torque & Flux calculator/1(V_abc)
  StatorIABC/1 -> Torque & Flux calculator/2(I_ABC)
  Data Type Conversion5/1 -> Gain/1
  Gain/1 -> Sum3/3
  Logical Operator/1 -> Data Type Conversion5/1
  dTe/2/1 -> Sum3/1, Logical Operator/1
  Sum1/1 -> -dTe/2/1, dTe/2/1
  -dTe/2/1 -> Logical Operator/2, Sum3/2
  PID Controller/1 -> Sum1/1
  RotorSpeed(rpm)/1 -> Flux table/1(|N|), Sum/2

== system BLDC_system_diagram/Field Oriented Controller/Field Oriented Control Current and Speed Controller ==
  note: void writestate (int sa, int sb, int sc)
      | {
      |   if (sa==1)    {digitalWrite(PhaseaUpperPin, HIGH);digitalWrite(PhaseaLowerPin, LOW);}
      |   if (sa==(-1)){digitalWrite(PhaseaUpperPin, LOW) ;digitalWrite(PhaseaLowerPin, HIGH);}
      |   if (sa==0)    {digitalWrite(PhaseaUpperPin, LOW) ;digitalWrite(PhaseaLowerPin, LOW);}
      |   if (sb==1)    {digitalWrite(PhasebUpperPin, HIGH);digitalWrite(PhasebLowerPin, LOW);}
      |   if (sb==(-1)){digitalWrite(PhasebUpperPin, LOW) ;digitalWrite(PhasebLowerPin, HIGH);}
      |   if (sb==0)    {digitalWrite(PhasebUpperPin, LOW) ;digitalWrite(PhasebLowerPin, LOW);}
      |   if (sc==1)    {digitalWrite(PhasecUpperPin, HIGH);digitalWrite(PhasecLowerPin, LOW);}
      |   if (sc==(-1)){digitalWrite(PhasecUpperPin, LOW) ;digitalWrite(PhasecLowerPin, HIGH);}
      |   if (sc==0)    {digitalWrite(PhasecUpperPin, LOW) ;digitalWrite(PhasecLowerPin, LOW);}
      | }
      |
      | void loop()
      | {
      |   Speedref=analogRead(SpeedrefPin);
      |   SpeedErrorOld=SpeedErrorNew;
      |   SpeedErrorNew=newspeed-Speedref;
      |   Iqref=kps*SpeedErrorNew+kis*(0.5)*(SpeedErrorNew+SpeedErrorOld)*Ts;
      |   Idref=0;
      |   I0ref=0;
      |
      |   IA=analogRead(IaPin);
      |   IB=analogRead(IbPin);
      |   IC=analogRead(IcPin);
      |
      |   Id=(2/3)*((1)  *IA+(-1/2)     *IB+(-1/2)      *IC);
      |   Iq=(2/3)*((0)  *IA+(sqrt(3)/2)*IB+(-sqrt(3)/2)*IC);
      |   I0=(2/3)*((1/2)*IA+(1/2)      *IB+(1/2)       *IC);
      |
      |   IAref=(1)   *(Idref*cos(thetae)-Iqref*sin(thetae))+(0)         *(Idref*sin(thetae)+Iqref*cos(thetae))+(1)*I0;
      |   IBref=(-1/2)*(Idref*cos(thetae)-Iqref*sin(thetae))+(sqrt(3)/2) *(Idref*sin(thetae)+Iqref*cos(thetae))+(1)*I0;
      |   ICref=(-1/2)*(Idref*cos(thetae)-Iqref*sin(thetae))+(-sqrt(3)/2)*(Idref*sin(thetae)+Iqref*cos(thetae))+(1)*I0;
      |
      |   gatesignal=B000;
      |   if (IAref-IA>tolerance){gatesignal|=(1<<2);}
      |   if (-IAref+IA>tolerance){gatesignal|=(0<<2);}
      |   if (IBref-IB>tolerance){gatesignal|=(1<<1);}
      |   if (-IBref+IB>tolerance){gatesignal|=(0<<1);}
      |   if (ICref-IC>tolerance){gatesignal|=(1<<0);}
      |   if (-ICref+IC>tolerance){gatesignal|=(0<<0);}
      |   writeState(gatesignal);delayMicroseconds(Ts);
      | }
  note: iabc
  note: idq0
  note: i0ref
  note: idref
  Stator IABC : Inport
  RotorSpeed(rpm) : Inport  Port=2
  Rotor Electrical Angle : Inport  Port=3
  ReferenceRotorSpeed(rpm) : Inport  Port=4
  Current Controller : Subsystem
  Mux1 : Mux  Inputs=3
  PID Controller : simulink/Continuous/PID Controller  Controller=PID  TimeDomain=Continuous-time  SampleTime=1  IntegratorMethod=Forward Euler  FilterMethod=Forward Euler  Form=Parallel  P=1  I=10  D=0  N=100  InitialConditionSource=internal  InitialConditionForIntegrator=0  InitialConditionForFilter=0  ExternalReset=none  LimitOutput=on  UpperSaturationLimit=100  LowerSaturationLimit=-100  LinearizeAsGain=on  AntiWindupMode=clamping  Kb=1  TrackingMode=off  Kt=1  PParamMin=[]  PParamMax=[]  IParamMin=[]  IParamMax=[]  DParamMin=[]  DParamMax=[]  NParamMin=[]  NParamMax=[]  KbParamMin=[]  KbParamMax=[]  KtParamMin=[]  KtParamMax=[]  POutMin=[]  POutMax=[]  IOutMin=[]  IOutMax=[]  DOutMin=[]  DOutMax=[]  NOutMin=[]  NOutMax=[]  KbOutMin=[]  KbOutMax=[]  KtOutMin=[]  KtOutMax=[]  IntegratorOutMin=[]  IntegratorOutMax=[]  FilterOutMin=[]  FilterOutMax=[]  SumOutMin=[]  SumOutMax=[]  SumI1OutMin=[]  SumI1OutMax=[]  SumI2OutMin=[]  SumI2OutMax=[]  SumI3OutMin=[]  SumI3OutMax=[]  SumDOutMin=[]  SumDOutMax=[]  SaturationOutMin=[]  SaturationOutMax=[]  IntegratorContinuousStateAttributes=''  IntegratorStateMustResolveToSignalObject=off  IntegratorRTWStateStorageClass=Auto  FilterContinuousStateAttributes=''  FilterStateMustResolveToSignalObject=off  FilterRTWStateStorageClass=Auto
  Sum2 : Sum  Inputs=+-|
  dq0 to abc : powerlib_meascontrol/Transformations/dq0 to abc  Alignment=Aligned with phase A axis
  i0ref : Constant  Value=0
  Gatings : Outport
  wires:
  RotorSpeed(rpm)/1 -> Sum2/2
  Sum2/1 -> PID Controller/1
  Mux1/1 -> dq0 to abc/1
  Stator IABC/1 -> Current Controller/2(Iabc)
  ReferenceRotorSpeed(rpm)/1 -> Sum2/1
  PID Controller/1 -> Mux1/2  "iqref"
  i0ref/1 -> Mux1/1, Mux1/3
  Rotor Electrical Angle/1 -> dq0 to abc/2
  dq0 to abc/1 -> Current Controller/1(Iabc_ref)
  Current Controller/1(Pulses) -> Gatings/1

== system BLDC_system_diagram/Hysteresis Speed and Current Controller/Hysteresis Speed and Current Controller ==
  note: void writestate (int sa, int sb, int sc)
      | {
      |   if (sa==1)    {digitalWrite(PhaseaUpperPin, HIGH);digitalWrite(PhaseaLowerPin, LOW);}
      |   if (sa==(-1)){digitalWrite(PhaseaUpperPin, LOW) ;digitalWrite(PhaseaLowerPin, HIGH);}
      |   if (sa==0)    {digitalWrite(PhaseaUpperPin, LOW) ;digitalWrite(PhaseaLowerPin, LOW);}
      |   if (sb==1)    {digitalWrite(PhasebUpperPin, HIGH);digitalWrite(PhasebLowerPin, LOW);}
      |   if (sb==(-1)){digitalWrite(PhasebUpperPin, LOW) ;digitalWrite(PhasebLowerPin, HIGH);}
      |   if (sb==0)    {digitalWrite(PhasebUpperPin, LOW) ;digitalWrite(PhasebLowerPin, LOW);}
      |   if (sc==1)    {digitalWrite(PhasecUpperPin, HIGH);digitalWrite(PhasecLowerPin, LOW);}
      |   if (sc==(-1)){digitalWrite(PhasecUpperPin, LOW) ;digitalWrite(PhasecLowerPin, HIGH);}
      |   if (sc==0)    {digitalWrite(PhasecUpperPin, LOW) ;digitalWrite(PhasecLowerPin, LOW);}
      | }
      |
      | void loop()
      | {
      |
      |   Speedref=analogRead(SpeedrefPin);
      |   SpeedErrorOld=SpeedErrorNew;
      |   SpeedErrorNew=newspeed-Speedref;
      |   Iref=kps*SpeedErrorNew+kis*(0.5)*(SpeedErrorNew+SpeedErrorOld)*Ts;
      |
      |   IA=analogRead(IaPin);
      |   IB=analogRead(IbPin);
      |   IC=analogRead(IcPin);
      |
      |   if (newstate==B000){EMFA=0;EMFB=0;EMFC=0;}
      |   if (newstate==B001){EMFA=0;EMFB=-1;EMFC=1;}
      |   if (newstate==B010){EMFA=-1;EMFB=1;EMFC=0;}
      |   if (newstate==B011){EMFA=-1;EMFB=0;EMFC=1;}
      |   if (newstate==B100){EMFA=1;EMFB=0;EMFC=-1;}
      |   if (newstate==B101){EMFA=1;EMFB=-1;EMFC=0;}
      |   if (newstate==B110){EMFA=0;EMFB=1;EMFC=-1;}
      |   if (newstate==B111){EMFA=0;EMFB=0;EMFC=0;}
      |
      |   IAref=EMFA*Iref;
      |   IBref=EMFB*Iref;
      |   ICref=EMFC*Iref;
      |
      |   gatesignal=B000;
      |   if (IAref-IA>tolerance){gatesignal|=(1<<2);}
      |   if (-IAref+IA>tolerance){gatesignal|=(0<<2);}
      |   if (IBref-IB>tolerance){gatesignal|=(1<<1);}
      |   if (-IBref+IB>tolerance){gatesignal|=(0<<1);}
      |   if (ICref-IC>tolerance){gatesignal|=(1<<0);}
      |   if (-ICref+IC>tolerance){gatesignal|=(0<<0);}
      |   writeState(gatesignal);delayMicroseconds(Ts);
      | }
  note: Iref
  HALLABC : Inport
  StatorIABC : Inport  Port=2
  RotorSpeed(rpm) : Inport  Port=3
  ReferenceRotorSpeed(rpm) : Inport  Port=4
  Current Controller : Subsystem
  Decoder : Subsystem
  PID Controller : simulink/Continuous/PID Controller  Controller=PID  TimeDomain=Continuous-time  SampleTime=1  IntegratorMethod=Forward Euler  FilterMethod=Forward Euler  Form=Parallel  P=0.005  I=0.100  D=0  N=100  InitialConditionSource=internal  InitialConditionForIntegrator=0  InitialConditionForFilter=0  ExternalReset=none  LimitOutput=on  UpperSaturationLimit=100  LowerSaturationLimit=-100  LinearizeAsGain=on  AntiWindupMode=none  Kb=1  TrackingMode=off  Kt=1  PParamMin=[]  PParamMax=[]  IParamMin=[]  IParamMax=[]  DParamMin=[]  DParamMax=[]  NParamMin=[]  NParamMax=[]  KbParamMin=[]  KbParamMax=[]  KtParamMin=[]  KtParamMax=[]  POutMin=[]  POutMax=[]  IOutMin=[]  IOutMax=[]  DOutMin=[]  DOutMax=[]  NOutMin=[]  NOutMax=[]  KbOutMin=[]  KbOutMax=[]  KtOutMin=[]  KtOutMax=[]  IntegratorOutMin=[]  IntegratorOutMax=[]  FilterOutMin=[]  FilterOutMax=[]  SumOutMin=[]  SumOutMax=[]  SumI1OutMin=[]  SumI1OutMax=[]  SumI2OutMin=[]  SumI2OutMax=[]  SumI3OutMin=[]  SumI3OutMax=[]  SumDOutMin=[]  SumDOutMax=[]  SaturationOutMin=[]  SaturationOutMax=[]  IntegratorContinuousStateAttributes=''  IntegratorStateMustResolveToSignalObject=off  IntegratorRTWStateStorageClass=Auto  FilterContinuousStateAttributes=''  FilterStateMustResolveToSignalObject=off  FilterRTWStateStorageClass=Auto
  Product : Product
  Sum : Sum  Inputs=|+-
  Gatings : Outport
  wires:
  PID Controller/1 -> Product/1
  Sum/1 -> PID Controller/1
  StatorIABC/1 -> Current Controller/2(Iabc)
  HALLABC/1 -> Decoder/1("Hall ")
  RotorSpeed(rpm)/1 -> Sum/2
  Decoder/1(Hall_abc) -> Product/2
  Current Controller/1(Pulses) -> Gatings/1
  Product/1 -> Current Controller/1(Iabc_ref)
  ReferenceRotorSpeed(rpm)/1 -> Sum/1

== system BLDC_system_diagram/Measurement System/Idq0 Calculator ==
  note: =
  note: [Id]
      | [Iq]
  note: [Ialpha]
      | [Ibeta]
  note: [cos(wt)   sin(wt)]
      | [-sin(wt)  cos(wt)]
  note: [Ia]
      | [Ib]
      | [Ic]
  note: [Ialpha]
      | [Ibeta]
      | [I0]
  note: =(2/3)
  note: [   1                  -1/2              -1/2]
      | [      0       sqrt(3)/2     -sqrt(3)/2  ]
      | [    1/2              1/2             1/2   ]
  Thetae : Inport
  IABC : Inport  Port=2
  abc to dq0 : powerlib_meascontrol/Transformations/abc to dq0  Alignment=Aligned with phase A axis
  Idq0 : Outport
  wires:
  IABC/1 -> abc to dq0/1
  Thetae/1 -> abc to dq0/2
  abc to dq0/1 -> Idq0/1

== system BLDC_system_diagram/Measurement System/Input Power Calculator ==
  note: PacInput=Va*Ia+Vb*Ib+Vc*Ic
  Vabc : Inport
  Iabc : Inport  Port=2
  Product : Product
  Sum of Elements : Sum  Inputs=+
  Pin : Outport
  wires:
  Vabc/1 -> Product/1
  Product/1 -> Sum of Elements/1
  Iabc/1 -> Product/2
  Sum of Elements/1 -> Pin/1

== system BLDC_system_diagram/Measurement System/Input Power Calculator1 ==
  note: PdcInput=Vdc*Idc
  Vdc : Inport
  Idc : Inport  Port=2
  Product : Product
  Pin : Outport
  wires:
  Vdc/1 -> Product/1
  Product/1 -> Pin/1
  Idc/1 -> Product/2

== system BLDC_system_diagram/Measurement System/Output Power Calculator ==
  note: PmOut=Torque*Speed(rad/s)
      | Speed(rad/s)=Speed(rpm)*(pi/30)
  Torque : Inport
  Speed : Inport  Port=2
  Gain : Gain  Gain=pi/30
  Product : Product
  Pout : Outport
  wires:
  Torque/1 -> Product/1
  Product/1 -> Pout/1
  Speed/1 -> Gain/1
  Gain/1 -> Product/2

== system BLDC_system_diagram/Measurement System/Speed, Acceleration, Direction and Angles Calculator ==
  note: Thetam=Thetae/Pole Pairs
      | P=Pole Pairs=Poles/2
  HALLABC : Inport
  Acceleration Calculator : Subsystem
  Clock and Direction : Subsystem
  Gain1 : Gain  Gain=1/P
  HALL change Detector : Subsystem
  Speed Calculator : Subsystem
  Subsystem : Subsystem
  delta Thetae Calculator : Subsystem
  Speed (rpm) : Outport
  Thetae : Outport  Port=2
  Direction : Outport  Port=3
  Thetaem : Outport  Port=4
  Acceleration : Outport  Port=5
  tag scope: Acceleration=global, Direction=global, Speed=global, Thetae=global
  wires:
  HALLABC/1 -> HALL change Detector/1(HALLABC)
  Clock and Direction/2(Clock) -> Speed Calculator/1(Clk)
  HALL change Detector/1(Change Detected) -> Clock and Direction/1(Change Detected)
  Clock and Direction/1(Direction) -> Direction/1, [Direction]
  Speed Calculator/2(New Clock Time) -> delta Thetae Calculator/2(Last Clock Time)
  Acceleration Calculator/1(Acceleration) -> [Acceleration], Acceleration/1
  Speed Calculator/1(Speed) -> delta Thetae Calculator/1(Speed (rpm)), Acceleration Calculator/1(Speed), Speed (rpm)/1, [Speed]
  HALL change Detector/2(Thetae0) -> Subsystem/1(Theta0)
  delta Thetae Calculator/1(dThetae) -> Subsystem/2(dTheta)
  Gain1/1 -> Thetaem/1
  Subsystem/1(Thetae) -> Thetae/1, Gain1/1, [Thetae]

== system BLDC_system_diagram/Measurement System/Subsystem ==
  Speed : Inport
  Add : Sum  Inputs=+-
  Compare To Zero1 : simulink/Logic and Bit Operations/Compare To Zero  relop=>=  OutDataTypeStr=boolean
  Constant : Constant  Value=0.5
  Gain1 : Gain  Gain=2
  Direction : Outport
  wires:
  Gain1/1 -> Direction/1
  Constant/1 -> Add/2
  Add/1 -> Gain1/1
  Compare To Zero1/1 -> Add/1
  Speed/1 -> Compare To Zero1/1

== system BLDC_system_diagram/Measurement System/Torque & Flux calculator ==
  note: phi_q = integral(vqs - iqs * Rs)
      | phi_d = integral(vds - ids * Rs)
      | phi=phi_q-j*phi_d
      | Flux Magnitude=|phi|=sqrt(phi_q*phi_q+phi_d*phi_d)
      | Flux Angle=atan(-phi_q/phi_d)*(180/pi)
      | Te=(3*P/2) * (phi_d * iqs - phi_q * ids)
      | P=Pole Pairs =Poles/2
  note: phi_d
  note: phi_q
  VABC : Inport
  IABC : Inport  Port=2
  Complex to Magnitude-Angle : ComplexToMagnitudeAngle
  Fcn : Fcn  Expr=u(1)
  Fcn1 : Fcn  Expr=u(2)
  Gain : Gain  Gain=Rss  SaturateOnIntegerOverflow=on  OutDataTypeStr=Inherit: Same as input  ParamDataTypeStr=Inherit: Same as input
  Gain1 : Gain  Gain=Rss  SaturateOnIntegerOverflow=on  OutDataTypeStr=Inherit: Same as input  ParamDataTypeStr=Inherit: Same as input
  Gain2 : Gain  Gain=3/2*P  SaturateOnIntegerOverflow=on  OutDataTypeStr=Inherit: Same as input  ParamDataTypeStr=Inherit: Same as input
  Gain5 : Gain  Gain=-1  SaturateOnIntegerOverflow=on  OutDataTypeStr=Inherit: Same as input  ParamDataTypeStr=Inherit: Same as input
  Mux : Mux  Inputs=2
  Product : Product  SaturateOnIntegerOverflow=on  OutDataTypeStr=Inherit: Same as first input
  Product1 : Product  SaturateOnIntegerOverflow=on  OutDataTypeStr=Inherit: Same as first input
  Rad2Deg : Gain  Gain=180/pi  SaturateOnIntegerOverflow=on  OutDataTypeStr=Inherit: Same as input  ParamDataTypeStr=Inherit: Same as input
  Real-Imag to Complex : RealImagToComplex
  Sum : Sum  Inputs=|+-  SaturateOnIntegerOverflow=on
  Sum1 : Sum  Inputs=|+-  SaturateOnIntegerOverflow=on
  Sum3 : Sum  Inputs=-+  SaturateOnIntegerOverflow=on
  Zero-Order Hold1 : ZeroOrderHold  SampleTime=Ts
  Zero-Order Hold2 : ZeroOrderHold  SampleTime=Ts
  Zero-Order Hold3 : ZeroOrderHold  SampleTime=Ts
  dq_I_transform : Subsystem
  dq_V_transform : Subsystem
  phi_d : DiscreteIntegrator  IntegratorMethod=Integration: Trapezoidal  SampleTime=Ts  ICPrevOutput=DiscIntNeverNeededParam  ICPrevScaledInput=DiscIntNeverNeededParam
  phi_q : DiscreteIntegrator  IntegratorMethod=Integration: Trapezoidal  SampleTime=Ts  ICPrevOutput=DiscIntNeverNeededParam  ICPrevScaledInput=DiscIntNeverNeededParam
  Torque : Outport
  Flux : Outport  Port=2
  angle : Outport  Port=3
  wires:
  Zero-Order Hold3/1 -> angle/1
  Zero-Order Hold1/1 -> Flux/1
  Zero-Order Hold2/1 -> Torque/1
  Product1/1 -> Sum3/2
  Gain5/1 -> Real-Imag to Complex/2
  Rad2Deg/1 -> Zero-Order Hold3/1
  Complex to Magnitude-Angle/2 -> Rad2Deg/1
  Complex to Magnitude-Angle/1 -> Zero-Order Hold1/1
  Real-Imag to Complex/1 -> Complex to Magnitude-Angle/1
  VABC/1 -> dq_V_transform/1(Vabc)
  dq_V_transform/1(v_q) -> Sum/1
  dq_I_transform/1(I_q) -> Gain/1, Product1/2  "i_qs"
  Gain/1 -> Sum/2
  Sum/1 -> phi_q/1
  dq_V_transform/2(v_d) -> Sum1/1
  Gain1/1 -> Sum1/2
  dq_I_transform/2(I_d) -> Product/2, Gain1/1  "i_ds"
  Sum1/1 -> phi_d/1
  phi_q/1 -> Real-Imag to Complex/1, Product/1
  phi_d/1 -> Gain5/1, Product1/1
  Product/1 -> Sum3/1
  Sum3/1 -> Gain2/1
  Gain2/1 -> Zero-Order Hold2/1
  IABC/1 -> Fcn1/1, Fcn/1
  Mux/1 -> dq_I_transform/1(I_ab)
  Fcn/1 -> Mux/1
  Fcn1/1 -> Mux/2
